simulink model "Lab1Part3"  (R2017b)
settings: Solver=ode4  StartTime=0.0  StopTime=1  FixedStep=1e-5  MaxStep=1e-4  RelTol=1e-4
libraries: powerlib x19, powerlib_meascontrol x4
settings Model: Creator=lwwang  LastModifiedBy=lwwang
settings CodeAppCC: StateflowObjectComments=on

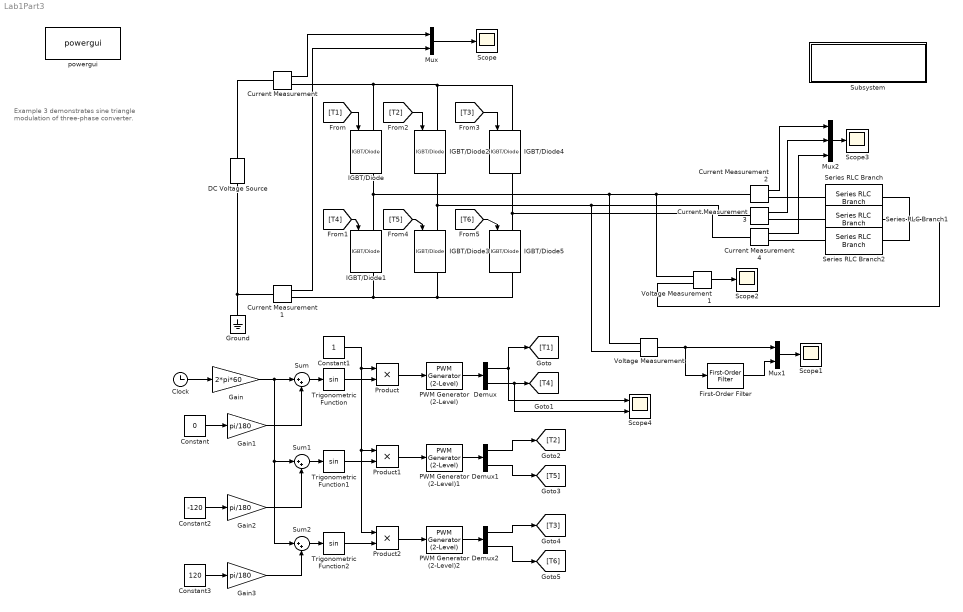
== system Lab1Part3 ==
  note: Example 3 demonstrates sine triangle modulation of three-phase converter.
  Clock : Clock
  Constant : Constant  Value=0
  Constant1 : Constant
  Constant2 : Constant  Value=-120
  Constant3 : Constant  Value=120
  Current Measurement{,1..4} (5 alike) : powerlib/Measurements/Current Measurement  PhasorSimulation=off  OutputType=Complex  PSBequivalent=0
  DC Voltage Source : powerlib/Electrical Sources/DC Voltage Source  Amplitude=1200  Measurements=None
  Demux : Demux  Outputs=2
  Demux1 : Demux  Outputs=2
  Demux2 : Demux  Outputs=2
  First-Order Filter : powerlib_meascontrol/Filters/First-Order Filter  FilterType=Lowpass  Tc=1e-3  Ts=0  Initialize=on  Vac_Init=[100, 0, 60]  Vdc_Init=0  PlotResponse=off  FreqRange="[0,  200,  1]"
      settings: SourceProductName=Simscape Power Systems
  Gain : Gain  Gain=2*pi*60
  Gain1 : Gain  Gain=pi/180
  Gain2 : Gain  Gain=pi/180
  Gain3 : Gain  Gain=pi/180
  Ground : powerlib/Elements/Ground  LConnTagsString=a
  IGBT/Diode{,1..5} (6 alike) : powerlib/Power Electronics/IGBT//Diode  Ron=1e-5  Rs=1e5  Cs=inf  Measurements=on
  Mux : Mux  Inputs=2
  Mux1 : Mux  Inputs=2
  Mux2 : Mux  Inputs=3
  PWM Generator (2-Level) : powerlib_meascontrol/Pulse & Signal Generators/PWM Generator (2-Level)  ModulatorType=Single-phase half-bridge (2 pulses)  ModulatorMode=Unsynchronized  Fc=1620  Pc=90  nF=30  MinMax="[ -1  1 ]"  SamplingTechnique=Natural  ModulatingSignals=off  m=0.8  Freq=60  Phase=0  Ts=1e-5  ShowCarrierOutport=off
      settings: SourceProductName=Simscape Power Systems
  PWM Generator (2-Level)1 : powerlib_meascontrol/Pulse & Signal Generators/PWM Generator (2-Level)  ModulatorType=Single-phase half-bridge (2 pulses)  ModulatorMode=Unsynchronized  Fc=1620  Pc=90  nF=30  MinMax="[ -1  1 ]"  SamplingTechnique=Natural  ModulatingSignals=off  m=0.8  Freq=60  Phase=0  Ts=1e-5  ShowCarrierOutport=off
      settings: SourceProductName=Simscape Power Systems
  PWM Generator (2-Level)2 : powerlib_meascontrol/Pulse & Signal Generators/PWM Generator (2-Level)  ModulatorType=Single-phase half-bridge (2 pulses)  ModulatorMode=Unsynchronized  Fc=1620  Pc=90  nF=30  MinMax="[ -1  1 ]"  SamplingTechnique=Natural  ModulatingSignals=off  m=0.8  Freq=60  Phase=0  Ts=1e-5  ShowCarrierOutport=off
      settings: SourceProductName=Simscape Power Systems
  Product : Product
  Product1 : Product
  Product2 : Product
  Scope{,1..3} (4 alike) : Scope
  Scope4 : Scope  NumInputPorts=2
  Series RLC Branch : powerlib/Elements/Series RLC Branch  LConnTagsString=__new0  RConnTagsString=__new0  BranchType=RL  Resistance=5  Inductance=0.5  SetiL0=off  InitialCurrent=0  Capacitance=1e-6  Setx0=off  InitialVoltage=0  Measurements=None
  Series RLC Branch1 : powerlib/Elements/Series RLC Branch  LConnTagsString=__new0  RConnTagsString=__new0  BranchType=RL  Resistance=5  Inductance=0.5  SetiL0=off  InitialCurrent=0  Capacitance=1e-6  Setx0=off  InitialVoltage=0  Measurements=None
  Series RLC Branch2 : powerlib/Elements/Series RLC Branch  LConnTagsString=__new0  RConnTagsString=__new0  BranchType=RL  Resistance=5  Inductance=0.5  SetiL0=off  InitialCurrent=0  Capacitance=1e-6  Setx0=off  InitialVoltage=0  Measurements=None
  Subsystem : Subsystem
      settings: OpenFcn=open_system('power_new_palette')
      mask Display: disp(sprintf('Open Simscape Power Systems\n(Specialized Technology)\nPalette Library'));
  Sum : Sum  Inputs=|++
  Sum1 : Sum  Inputs=|++
  Sum2 : Sum  Inputs=|++
  Trigonometric Function : Trigonometry
  Trigonometric Function1 : Trigonometry
  Trigonometric Function2 : Trigonometry
  Voltage Measurement : powerlib/Measurements/Voltage Measurement  PhasorSimulation=off  OutputType=Complex  PSBequivalent=0
  Voltage Measurement1 : powerlib/Measurements/Voltage Measurement  PhasorSimulation=off  OutputType=Complex  PSBequivalent=0
  powergui : powerlib/powergui  Priority=1  SimulationMode=Discrete  SampleTime=1e-5  frequency=60  Iterations=50  frequencyindice=0  Pbase=100e6  ErrMax=1e-4  UnitsV=kV  UnitsW=MW  buscounter=0  FunctionMessages=off  echomessages=off  EnableUseOfTLC=off  CurrentSourceSwitches=off  DisableSnubberDevices=off  DisableRonSwitches=off  DisableVfSwitches=off  DisplayEquations=off  SolverType=Tustin/Backward Euler (TBE)  Interpol=off  ExternalGateDelay=off  methode=off  Ts=100  x0status=blocks  SPID=on  SwTol=0  HookPort=off  RestoreLinks=warning  ResistiveCurrentMeasurement=off  Frange=[0:2:500]  Ylog=off  Xlog=on  ShowGrid=off  save=off  variable=ZData  structure=0  ZoomFFT=off  StartTime=0.0  cycles=1  DisplayStyle=1  fundamental=60  FreqAxis=off  MaxFrequency=1000  frequencyindicesteady=1  RmsSteady=1  display=off
  wires:
  Clock/1 -> Gain/1
  Gain/1 -> Sum2/1, Sum1/1, Sum/1
  Constant/1 -> Gain1/1
  Sum/1 -> Trigonometric Function/1
  Gain1/1 -> Sum/2
  PWM Generator (2-Level)/1 -> Demux/1
  Mux/1 -> Scope/1
  Current Measurement/1 -> Mux/1
  Current Measurement1/1 -> Mux/2
  Mux1/1 -> Scope1/1
  Voltage Measurement/1 -> Mux1/1, First-Order Filter/1
  Trigonometric Function/1 -> Product/2
  Constant1/1 -> Product2/1, Product1/1, Product/1
  Product/1 -> PWM Generator (2-Level)/1
  First-Order Filter/1 -> Mux1/2
  Constant2/1 -> Gain2/1
  Gain2/1 -> Sum1/2
  Sum1/1 -> Trigonometric Function1/1
  Trigonometric Function1/1 -> Product1/2
  Product1/1 -> PWM Generator (2-Level)1/1
  Gain3/1 -> Sum2/2
  Constant3/1 -> Gain3/1
  Sum2/1 -> Trigonometric Function2/1
  Trigonometric Function2/1 -> Product2/2
  Product2/1 -> PWM Generator (2-Level)2/1
  PWM Generator (2-Level)1/1 -> Demux1/1
  PWM Generator (2-Level)2/1 -> Demux2/1
  [T2] -> IGBT/Diode2/1
  [T1] -> IGBT/Diode/1
  [T4] -> IGBT/Diode1/1
  Demux1/1 -> [T2]
  Demux1/2 -> [T5]
  Demux2/1 -> [T3]
  Demux2/2 -> [T6]
  [T3] -> IGBT/Diode4/1
  [T5] -> IGBT/Diode3/1
  [T6] -> IGBT/Diode5/1
  Voltage Measurement1/1 -> Scope2/1
  Demux/2 -> Scope4/2, [T4]
  Demux/1 -> Scope4/1, [T1]
  Mux2/1 -> Scope3/1
  Current Measurement2/1 -> Mux2/1
  Current Measurement3/1 -> Mux2/2
  Current Measurement4/1 -> Mux2/3
  connections:
  Series RLC Branch/RConn1 -- Voltage Measurement1/LConn2 -- Series RLC Branch2/RConn1 -- Series RLC Branch1/RConn1
  Current Measurement2/LConn1 -- IGBT/Diode1/LConn1 -- IGBT/Diode/RConn1 -- Voltage Measurement/LConn1 -- Voltage Measurement1/LConn1
  IGBT/Diode/LConn1 -- IGBT/Diode4/LConn1 -- IGBT/Diode2/LConn1 -- Current Measurement/RConn1
  Current Measurement/LConn1 -- DC Voltage Source/RConn1
  DC Voltage Source/LConn1 -- Current Measurement1/LConn1 -- Ground/LConn1
  Current Measurement1/RConn1 -- IGBT/Diode5/RConn1 -- IGBT/Diode3/RConn1 -- IGBT/Diode1/RConn1
  Current Measurement2/RConn1 -- Series RLC Branch/LConn1
  IGBT/Diode3/LConn1 -- Current Measurement3/LConn1 -- Voltage Measurement/LConn2 -- IGBT/Diode2/RConn1
  IGBT/Diode5/LConn1 -- Current Measurement4/LConn1 -- IGBT/Diode4/RConn1
  Current Measurement3/RConn1 -- Series RLC Branch1/LConn1
  Current Measurement4/RConn1 -- Series RLC Branch2/LConn1

== system Lab1Part3/Subsystem ==
